simulink model "TricopterModel"  (R2015a)
settings: Solver=ode3  SolverMode=SingleTasking  StartTime=0.0  StopTime=10.0  FixedStep=T_sim  RelTol=1e-3
values from neighbouring files (symbols this model uses):
  a = 10.26    [SetupComplete.m]
  A_x = 0.015    [SetupComplete.m]
  A_y = A_x    (= 0.015)    [SetupComplete.m]
  A_z = 0.16    [SetupComplete.m]
  C_d0 = 0.001193    [SetupComplete.m]
  C_x = 1.2    [SetupComplete.m]
  C_y = C_x    (= 1.2)    [SetupComplete.m]
  C_z = 2.2    [SetupComplete.m]
  CG_0 = [0,0,0.02]'    [SetupComplete.m]
  eta_23 = deg2rad(-1.42)    [Run3Copter.m]
  h = 0.08    [SetupComplete.m]
  h_M = 0.064    [SetupComplete.m]
  I_BAC_0 = [ Ix,0,Ixz;0,Iy,0;Ixz,0,Iz]    [SetupComplete.m]
  Initial_Omegas = [1;1;1]*Omega_hover    [Run3Copter.m]
  l = 0.3450    (= 0.345)    [NDI_components.m]    (also in SetupComplete.m; robust_controller.m)
  l_arm = 0.264    [SetupComplete.m]
  m = 3.51    [SetupComplete.m]
  m_0 = 2.61    [SetupComplete.m]
  m_M = 0.300    (= 0.3)    [SetupComplete.m]
  R = 0.1778    [SetupComplete.m]    (also in robust_controller.m = eye(4))
  rho = 1.15    [SetupComplete.m]
  Rotation_sign = [ 1,-1,-1]    [SetupComplete.m]
  sigma = b*c/(pi*R)    (= 0.107416159567)    [SetupComplete.m]
  theta_0 = 0.38397    [SetupComplete.m]
  theta_1 = -0.2967    [SetupComplete.m]
  v_i0 = sqrt( 1/3*m*g/(2*rho*pi*R^2)  )    [SetupComplete.m]
undefined symbols (not defined in the file or in its folder): DOWN_0, EAST_0, Motor, NORTH_0, P_0, Prop, Q_0, R_0, Throttle_Hover, U_0, V_0, v_i_adim, Vx_adim, Vz_adim, W_0
undefined symbols (not defined in the file): Initial_Torques, J_FA, J_T, Tau_motors
libraries: XXCopter x22, simulink_extras x7, vrlib x6, XXCopter_C x3, aerolibutil x2, aerolib6dofsys x1
(part 1 of 2)
settings Model: ExtModeTrigDuration=5000  Creator=DavidTorres  LastModifiedBy=juan
settings OptimizationCC: BlockReduction=off  BooleanDataType=off
settings DebuggingCC: SaveWithParameterizedLinksMsg=none  UnderspecifiedInitializationDetection=Classic  MergeDetectMultiDrivingBlocksExec=none  SignalResolutionControl=TryResolveAllWithWarning
settings HardwareCC: TargetUnknown=on

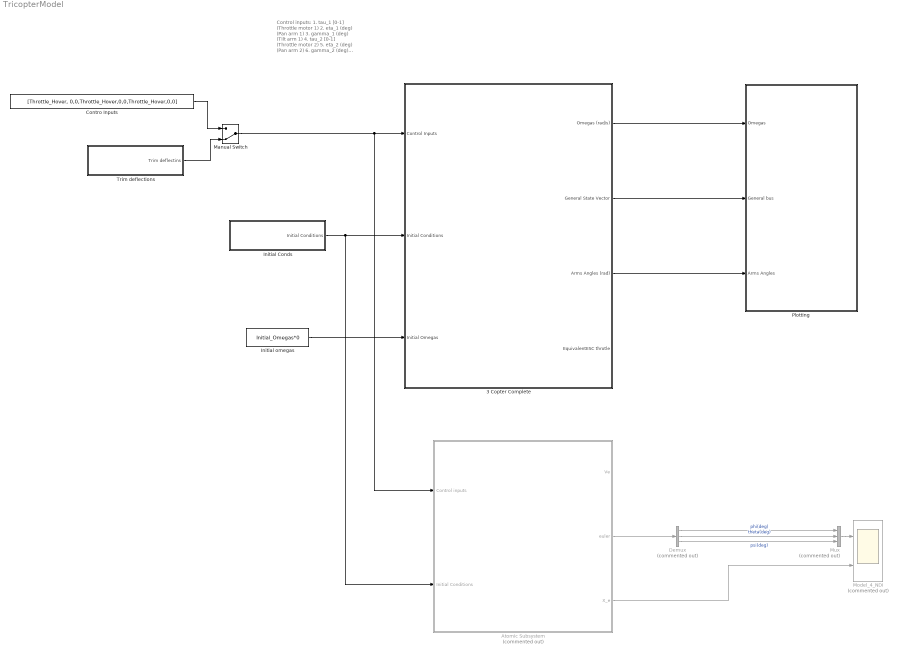
== system TricopterModel ==
  note: Control inputs:
      | 1. tau_1 [0-1] (Throttle motor 1)
      | 2. eta_1 (deg)  (Pan arm 1)
      | 3. gamma_1 (deg)  (Tilt arm 1)
      |
      | 4. tau_2 [0-1] (Throttle motor 2)
      | 5. eta_2 (deg)  (Pan arm 2)
      | 6. gamma_2 (deg)  (Tilt arm 2)
      |
      | 7. tau_3 [0-1] (Throttle motor 3)
      | 8. eta_3 (deg)  (Pan arm  3)
      | 9. gamma_3 (deg)  (Tilt arm 3)
  3 Copter Complete : Subsystem
  Atomic Subsystem : Subsystem  Commented=on
  Contro Inputs : Constant  Value=[Throttle_Hover, 0,0,Throttle_Hover,0,0,Throttle_Hover,0,0]
  Demux : Demux  Commented=on  Outputs=3
  Initial Conds : Subsystem  TreatAsAtomicUnit=on
  Initial omegas : Constant  Value=Initial_Omegas*0
  Manual Switch : ManualSwitch  CurrentSetting=0
  Model_4_NDI : Scope  Commented=on  NumInputPorts=2
      settings: ShowLegends=on  YMin=-5e-05~-21  YMax=0.00045~1  SaveName=ScopeData3
  Mux : Mux  Commented=on  Inputs=3
  Plotting : Subsystem
  Trim deflections : Subsystem  TreatAsAtomicUnit=on
  wires:
  Initial omegas/1 -> 3 Copter Complete/3(Initial Omegas)
  Initial Conds/1(Initial Conditions) -> Atomic Subsystem/2(Initial Conditions), 3 Copter Complete/2(Initial Conditions)
  3 Copter Complete/2(General State Vector) -> Plotting/2(General bus)
  3 Copter Complete/1(Omegas (rad/s)) -> Plotting/1(Omegas)
  3 Copter Complete/3(Arms Angles (rad)) -> Plotting/3(Arms Angles)
  Manual Switch/1 -> 3 Copter Complete/1(Control Inputs), Atomic Subsystem/1(Control inputs)
  Contro Inputs/1 -> Manual Switch/1
  Trim deflections/1(Trim deflectins) -> Manual Switch/2
  Atomic Subsystem/2(euler) -> Demux/1
  Demux/3 -> Mux/3  "psi(deg)"
  Demux/1 -> Mux/1  "phi(deg)"
  Demux/2 -> Mux/2  "theta(deg)"
  Mux/1 -> Model_4_NDI/1
  Atomic Subsystem/3(X_e) -> Model_4_NDI/2

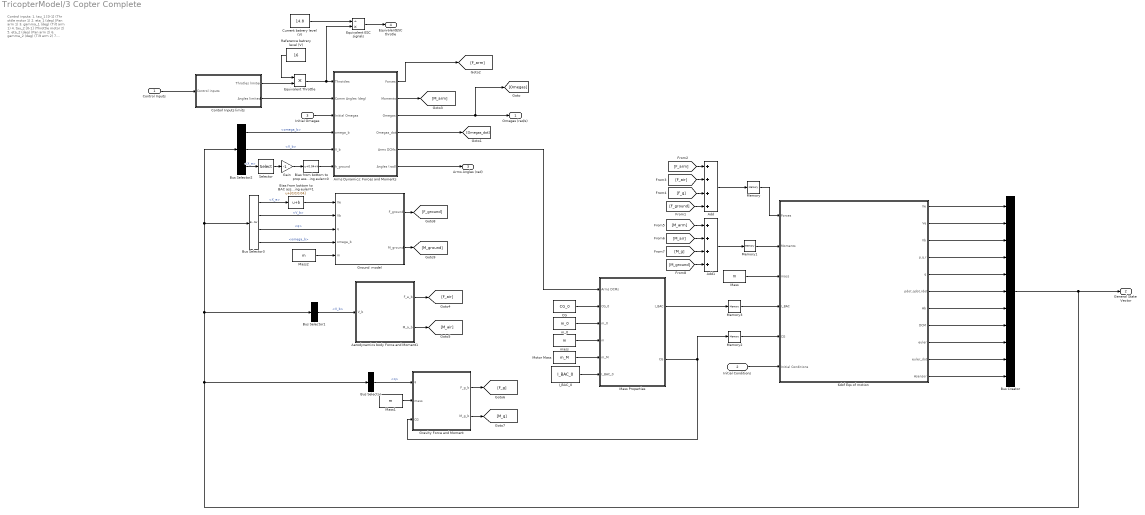
== system TricopterModel/3 Copter Complete ==
  note: Control inputs:
      | 1. tau_1 [0-1] (Thr ottle motor 1)
      | 2. eta_1 (deg)  (Pan arm 1)
      | 3. gamma_1 (deg)  (Tilt arm 1)
      |
      | 4. tau_2 [0-1] (Throttle motor 2)
      | 5. eta_2 (deg)  (Pan arm 2)
      | 6. gamma_2 (deg)  (Tilt arm 2)
      |
      | 7. tau_3 [0-1] (Throttle motor 3)
      | 8. eta_3 (deg)  (Pan arm  3)
      | 9. gamma_3 (deg)  (Tilt arm 3)
  Control Inputs : Inport
  Initial Conditions : Inport  Port=2
  Initial Omegas : Inport  Port=3
  6dof Eqs of motion : Subsystem  TreatAsAtomicUnit=on
  Add : Sum  Inputs=++++
  Add1 : Sum  Inputs=++++
  Aerodynamics body Force and Moment1 : MATLAB Function  TreatAsAtomicUnit=on
  Arms Dynamics: Forces and Moments : Subsystem
  Bias from bottom to BAC assuming euler=1 : Bias  Bias=[0;0;0.04]
  Bias from bottom to prop assuming euler=0 : Bias  Bias=0.04+h
  Bus Creator : BusCreator  Inputs=11
  Bus Selector : BusSelector  OutputSignals=q
  Bus Selector1 : BusSelector  OutputSignals=V_b
  Bus Selector2 : BusSelector  OutputSignals=omega_b,V_b,X_e
  Bus Selector3 : BusSelector  OutputSignals=X_e,V_b,q,omega_b
  CG : Constant  Value=CG_0
  Contorl Inputs limits : Subsystem  TreatAsAtomicUnit=on
  Current batrery level (V) : Constant  Value=14.8
  Equivalent ESC signals : Product  Inputs=/*
  Equivalent Throttle : Product  Inputs=**
  Gain : Gain  Gain=-1
  Gravity Force and Moment : MATLAB Function  TreatAsAtomicUnit=on
  Ground  model : Subsystem  TreatAsAtomicUnit=on
  I_BAC_0 : Constant  Value=I_BAC_0
  Mass : Constant  Value=m
  Mass Properties : Subsystem  TreatAsAtomicUnit=on
  Mass1 : Constant  Value=m
  Mass2 : Constant  Value=m
  Memory : Memory  X0=[0,0,0]
  Memory1 : Memory  X0=[0,0,0]
  Memory2 : Memory  X0=CG_0
  Memory3 : Memory  X0=I_BAC_0
  Motor Mass : Constant  Value=m_M
  Reference batrery level (V) : Constant  Value=16
  Selector : Selector  InputPortWidth=3  Indices=3
  m_0 : Constant  Value=m_0
  mass : Constant  Value=m
  Omegas (rad/s) : Outport
  General State Vector : Outport  Port=2
  Arms Angles (rad) : Outport  Port=3
  EquivalentESC throtle : Outport  Port=4
  wires:
  Initial Conditions/1 -> 6dof Eqs of motion/6(Initial Conditions)
  6dof Eqs of motion/3(Vb) -> Bus Creator/3
  6dof Eqs of motion/5(q) -> Bus Creator/5
  6dof Eqs of motion/2(Ve) -> Bus Creator/2
  6dof Eqs of motion/6(pdot,qdot,rdot) -> Bus Creator/6
  6dof Eqs of motion/1(Xe) -> Bus Creator/1
  6dof Eqs of motion/7(Ab) -> Bus Creator/7
  6dof Eqs of motion/8(DCM) -> Bus Creator/8
  6dof Eqs of motion/9(euler) -> Bus Creator/9
  6dof Eqs of motion/10(euler_dot) -> Bus Creator/10
  Bus Selector/1 -> Gravity Force and Moment/1(q)  "<q>"
  Mass/1 -> 6dof Eqs of motion/3(mass)
  Mass Properties/1(I_BAC) -> Memory3/1
  Bus Selector1/1 -> Aerodynamics body Force and Moment1/1(V_b)  "<V_b>"
  Bus Selector2/1 -> Arms Dynamics: Forces and Moments/4(omega_b)  "<omega_b>"
  Bus Selector2/2 -> Arms Dynamics: Forces and Moments/5(V_b)  "<V_b>"
  Mass1/1 -> Gravity Force and Moment/2(mass)
  Mass Properties/2(CG) -> Gravity Force and Moment/3(CG), Memory2/1
  Arms Dynamics: Forces and Moments/4(Omegas_dot) -> [Omegas_dot]
  Initial Omegas/1 -> Arms Dynamics: Forces and Moments/3(Initial Omegas)
  Bus Selector2/3 -> Selector/1  "<X_e>"
  Selector/1 -> Gain/1
  Gain/1 -> Bias from bottom to prop assuming euler=0/1
  Add/1 -> Memory/1
  Add1/1 -> Memory1/1
  Arms Dynamics: Forces and Moments/1(Forces) -> [F_arm]
  Arms Dynamics: Forces and Moments/2(Moments) -> [M_arm]
  Aerodynamics body Force and Moment1/1(F_a_b) -> [F_air]
  Aerodynamics body Force and Moment1/2(M_a_b) -> [M_air]
  Gravity Force and Moment/1(F_g_b) -> [F_g]
  Gravity Force and Moment/2(M_g_b) -> [M_g]
  [F_arm] -> Add/1
  [F_air] -> Add/2
  [F_g] -> Add/3
  [M_arm] -> Add1/1
  [M_g] -> Add1/3
  [M_air] -> Add1/2
  6dof Eqs of motion/11(Asensor) -> Bus Creator/11
  Contorl Inputs limits/1(Throtles limited) -> Equivalent Throttle/2
  Contorl Inputs limits/2(Angles limited) -> Arms Dynamics: Forces and Moments/2(Comm Angles (deg))
  Arms Dynamics: Forces and Moments/5(Arms DCMs) -> Mass Properties/1(Arms DCMs)
  CG/1 -> Mass Properties/2(CG_0)
  Motor Mass/1 -> Mass Properties/5(m_M)
  I_BAC_0/1 -> Mass Properties/6(I_BAC_0)
  m_0/1 -> Mass Properties/3(m_0)
  mass/1 -> Mass Properties/4(m)
  Arms Dynamics: Forces and Moments/3(Omegas) -> [Omegas], Omegas (rad/s)/1
  Bus Creator/1 -> Bus Selector2/1, Bus Selector3/1, Bus Selector1/1, Bus Selector/1, General State Vector/1
  Memory/1 -> 6dof Eqs of motion/1(Forces)
  Memory1/1 -> 6dof Eqs of motion/2(Moments)
  Memory2/1 -> 6dof Eqs of motion/5(CG)
  Memory3/1 -> 6dof Eqs of motion/4(I_BAC)
  Equivalent Throttle/1 -> Equivalent ESC signals/2, Arms Dynamics: Forces and Moments/1(Throttles)
  Reference batrery level (V)/1 -> Equivalent Throttle/1
  Current batrery level (V)/1 -> Equivalent ESC signals/1
  Equivalent ESC signals/1 -> EquivalentESC throtle/1
  6dof Eqs of motion/4(p,q,r) -> Bus Creator/4
  Arms Dynamics: Forces and Moments/6(Angles (rad)) -> Arms Angles (rad)/1
  Control Inputs/1 -> Contorl Inputs limits/1(Control inputs)
  Bus Selector3/1 -> Bias from bottom to BAC assuming euler=1/1  "<X_e>"
  Bus Selector3/3 -> Ground  model/3(q)  "<q>"
  Ground  model/1(F_ground) -> [F_ground]
  Ground  model/2(M_ground) -> [M_ground]
  [F_ground] -> Add/4
  [M_ground] -> Add1/4
  Mass2/1 -> Ground  model/5(m)
  Bus Selector3/2 -> Ground  model/2(Vb)  "<V_b>"
  Bus Selector3/4 -> Ground  model/4(omega_b)  "<omega_b>"
  Bias from bottom to prop assuming euler=0/1 -> Arms Dynamics: Forces and Moments/6(h_ground)
  Bias from bottom to BAC assuming euler=1/1 -> Ground  model/1(Xe)

== system TricopterModel/Atomic Subsystem ==
  Control inputs : Inport
  Initial Conditions : Inport  Port=2
  3Copter_4_NDI : Subsystem
  Bus Selector : BusSelector  OutputSignals=X_e_0,V_e_0,Euler_0,Euler_dot_0
  Ground : Ground
  Ground1 : Ground
  Ground2 : Ground
  Normalize Quaternion : Subsystem  TreatAsAtomicUnit=on
  SVFI_to_SVFb : MATLAB Function  TreatAsAtomicUnit=on
  SV_F_b_to_SV_FI : MATLAB Function  TreatAsAtomicUnit=on
  "p,q,r " : Integrator  InitialConditionSource=external  InitialCondition=[P_0,Q_0,R_0]
  quaternion : Integrator  InitialConditionSource=external  InitialCondition=[P_0,Q_0,R_0]
  ub,vb,wb : Integrator  InitialConditionSource=external  InitialCondition=[U_0,V_0,W_0]
  xe,ye,ze : Integrator  InitialConditionSource=external  InitialCondition=[NORTH_0,EAST_0,-DOWN_0]
  Ve : Outport
  euler : Outport  Port=2
  X_e : Outport  Port=3
  wires:
  Initial Conditions/1 -> Bus Selector/1
  Bus Selector/1 -> SVFI_to_SVFb/1(X_e)  "<X_e_0>"
  Bus Selector/2 -> SVFI_to_SVFb/2(V_e)  "<V_e_0>"
  Bus Selector/3 -> SVFI_to_SVFb/3(Euler_Ang)  "<Euler_0>"
  Bus Selector/4 -> SVFI_to_SVFb/4(Euler_Ang_Dot)  "<Euler_dot_0>"
  3Copter_4_NDI/4(omega_b_dot) -> "p,q,r "/1
  SVFI_to_SVFb/4(omega_b) -> "p,q,r "/2
  3Copter_4_NDI/3(q_dot) -> quaternion/1
  SVFI_to_SVFb/3(q) -> quaternion/2
  quaternion/1 -> Normalize Quaternion/1(q)
  3Copter_4_NDI/2(Ab) -> ub,vb,wb/1
  SVFI_to_SVFb/2(V_b) -> ub,vb,wb/2
  3Copter_4_NDI/1(Ve) -> Ve/1, xe,ye,ze/1
  Control inputs/1 -> 3Copter_4_NDI/1(Control Inputs)
  SVFI_to_SVFb/1(X_e_out) -> xe,ye,ze/2
  xe,ye,ze/1 -> X_e/1, 3Copter_4_NDI/2(X_e)
  ub,vb,wb/1 -> 3Copter_4_NDI/3(Vb)
  Normalize Quaternion/1(normal(q)) -> SV_F_b_to_SV_FI/1(q), 3Copter_4_NDI/4(q)
  "p,q,r "/1 -> 3Copter_4_NDI/5(omega_b)
  Ground/1 -> 3Copter_4_NDI/6(Omegas_dot_actual)
  Ground1/1 -> 3Copter_4_NDI/7(angles_actual)
  Ground2/1 -> 3Copter_4_NDI/8(angles_dot_actual)
  SV_F_b_to_SV_FI/1(euler) -> euler/1  "euler"

== system TricopterModel/Initial Conds ==
  Bus Creator : BusCreator
  Ini Position X_e_0 : Constant  Value=[0;0;-1]
  Initial Attitude Euler_0 : Constant  Value=[deg2rad(0);deg2rad(0);deg2rad(0)]
  Initial Attitude Rate  Euler_dot_0 : Constant  Value=[deg2rad(0);deg2rad(0);deg2rad(0)]
  Initial Velocity V_e_0 : Constant  Value=[0;0;0]
  Initial Conditions : Outport
  wires:
  Ini Position X_e_0/1 -> Bus Creator/1  "X_e_0"
  Initial Velocity V_e_0/1 -> Bus Creator/2  "V_e_0"
  Initial Attitude Euler_0/1 -> Bus Creator/3  "Euler_0"
  Initial Attitude Rate  Euler_dot_0/1 -> Bus Creator/4  "Euler_dot_0"
  Bus Creator/1 -> Initial Conditions/1

== system TricopterModel/Plotting ==
  Omegas : Inport
  General bus : Inport  Port=2
  Arms Angles : Inport  Port=3
  Bus Selector : BusSelector  OutputSignals=euler,X_e,DCM
  Bus Selector1 : BusSelector  OutputSignals=Angles Arm 1,Angles Arm 2,Angles Arm 3
  Demux : Demux  Outputs=3
  Level-2 MATLAB S-Function : M-S-Function  FunctionName=Simulation_3_copter
  Mux : Mux  Inputs=3
  Scope : Scope  NumInputPorts=2
      settings: ShowLegends=on  YMin=-5e-05~-21  YMax=0.00045~1
  Scope1 : Scope
      settings: TimeRange=5  YMin=564.75  YMax=570
  Scope2 : Scope  NumInputPorts=3
      settings: ShowLegends=on  YMin=-5~-5~-5  YMax=5~5~5  SaveName=ScopeData2
  wires:
  General bus/1 -> Bus Selector/1
  Bus Selector/1 -> Demux/1  "<euler>"
  Omegas/1 -> Scope1/1  "Omegas"
  Arms Angles/1 -> Bus Selector1/1
  Bus Selector1/3 -> Level-2 MATLAB S-Function/8, Scope2/3  "<Angles Arm 3>"
  Bus Selector1/2 -> Level-2 MATLAB S-Function/7, Scope2/2  "<Angles Arm 2>"
  Bus Selector1/1 -> Level-2 MATLAB S-Function/6, Scope2/1  "<Angles Arm 1>"
  Bus Selector/2 -> Level-2 MATLAB S-Function/1, Scope/2  "<X_e>"
  [r_p_3] -> Level-2 MATLAB S-Function/5
  [r_p_2] -> Level-2 MATLAB S-Function/4
  [r_p_1] -> Level-2 MATLAB S-Function/3
  Bus Selector/3 -> Level-2 MATLAB S-Function/2  "<DCM>"
  Demux/3 -> Mux/3  "psi(deg)"
  Demux/1 -> Mux/1  "phi(deg)"
  Demux/2 -> Mux/2  "theta(deg)"
  Mux/1 -> Scope/1

== system TricopterModel/Trim deflections ==
  " " : simulink_extras/Transformations/Radians to Degrees
  Contro Inputs1 : Constant  Value=0
  Contro Inputs2 : Constant  Value=0
  Contro Inputs3 : Constant  Value=eta_23
  Gain : Gain  Gain=-1
  Ground : Ground
  Mux : Mux  Inputs=9
  Trim deflectins : Outport
  wires:
  Contro Inputs1/1 -> Mux/1
  Contro Inputs2/1 -> Mux/7, Mux/4
  Ground/1 -> Mux/2, Mux/6, Mux/9, Mux/3
  Contro Inputs3/1 -> " "/1
  " "/1 -> Gain/1, Mux/5
  Gain/1 -> Mux/8
  Mux/1 -> Trim deflectins/1

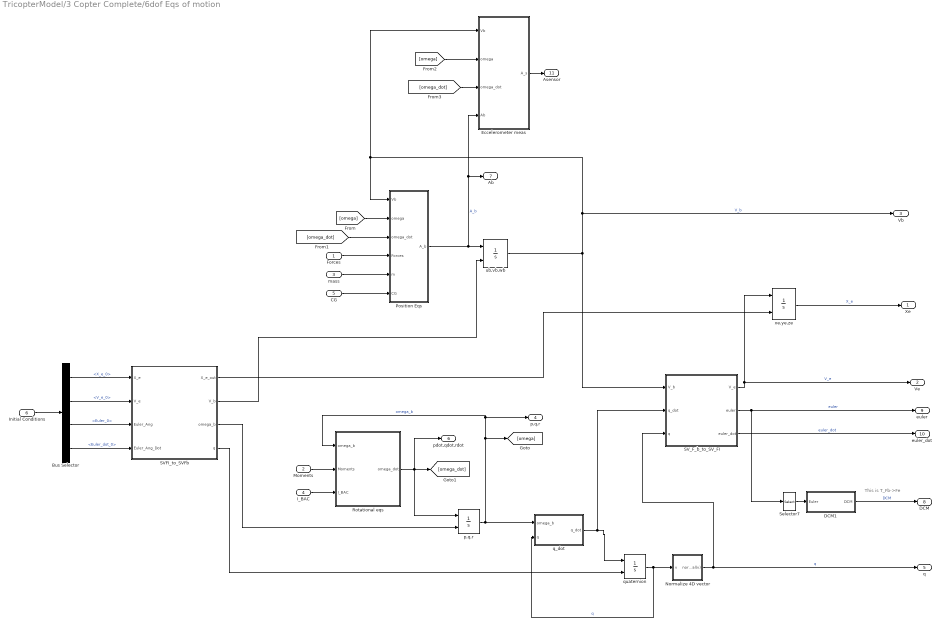
== system TricopterModel/3 Copter Complete/6dof Eqs of motion ==
  note: This is T_Fb->Fe
  Forces : Inport
  Moments : Inport  Port=2
  mass : Inport  Port=3
  I_BAC : Inport  Port=4
  CG : Inport  Port=5
  Initial Conditions : Inport  Port=6
  Bus Selector : BusSelector  OutputSignals=X_e_0,V_e_0,Euler_0,Euler_dot_0
  DCM1 : Subsystem  TreatAsAtomicUnit=on
  Eccelerometer meas : MATLAB Function  TreatAsAtomicUnit=on
  Normalize 4D vector : Subsystem  AncestorBlock=XXCopter/Normalize 4D vector  TreatAsAtomicUnit=on
  Position Eqs : MATLAB Function  TreatAsAtomicUnit=on
  Rotational eqs : MATLAB Function  TreatAsAtomicUnit=on
  SVFI_to_SVFb : MATLAB Function  TreatAsAtomicUnit=on
  SV_F_b_to_SV_FI : MATLAB Function  TreatAsAtomicUnit=on
  Selector7 : Selector  InputPortWidth=3  Indices=[3 2 1]
  "p,q,r " : Integrator  InitialConditionSource=external  InitialCondition=[P_0,Q_0,R_0]
  q_dot : Subsystem  TreatAsAtomicUnit=on
  quaternion : Integrator  InitialConditionSource=external  InitialCondition=[P_0,Q_0,R_0]
  ub,vb,wb : Integrator  InitialConditionSource=external  InitialCondition=[U_0,V_0,W_0]
  xe,ye,ze : Integrator  InitialConditionSource=external  InitialCondition=[NORTH_0,EAST_0,-DOWN_0]
  Xe : Outport
  Ve : Outport  Port=2
  Vb : Outport  Port=3
  p,q,r : Outport  Port=4
  q : Outport  Port=5
  pdot,qdot,rdot : Outport  Port=6
  Ab : Outport  Port=7
  DCM : Outport  Port=8
  euler : Outport  Port=9
  euler_dot : Outport  Port=10
  Asensor : Outport  Port=11
  wires:
  I_BAC/1 -> Rotational eqs/3(I_BAC)
  mass/1 -> Position Eqs/5(m)
  Forces/1 -> Position Eqs/4(Forces)
  xe,ye,ze/1 -> Xe/1  "X_e"
  ub,vb,wb/1 -> Vb/1, Eccelerometer meas/1(Vb), Position Eqs/1(Vb), SV_F_b_to_SV_FI/1(V_b)  "V_b"
  SV_F_b_to_SV_FI/1(V_e) -> Ve/1, xe,ye,ze/1  "V_e"
  [omega] -> Position Eqs/2(omega)
  [omega_dot] -> Position Eqs/3(omega_dot)
  Position Eqs/1(A_b) -> Eccelerometer meas/4(Ab), Ab/1, ub,vb,wb/1  "A_b"
  CG/1 -> Position Eqs/6(CG)
  Initial Conditions/1 -> Bus Selector/1
  Bus Selector/1 -> SVFI_to_SVFb/1(X_e)  "<X_e_0>"
  Bus Selector/2 -> SVFI_to_SVFb/2(V_e)  "<V_e_0>"
  Bus Selector/3 -> SVFI_to_SVFb/3(Euler_Ang)  "<Euler_0>"
  Bus Selector/4 -> SVFI_to_SVFb/4(Euler_Ang_Dot)  "<Euler_dot_0>"
  SVFI_to_SVFb/2(V_b) -> ub,vb,wb/2
  SVFI_to_SVFb/1(X_e_out) -> xe,ye,ze/2
  SVFI_to_SVFb/3(omega_b) -> "p,q,r "/2
  Rotational eqs/1(omega_dot) -> pdot,qdot,rdot/1, [omega_dot], "p,q,r "/1
  "p,q,r "/1 -> q_dot/1(omega_b), [omega], p,q,r/1, Rotational eqs/1(omega_b)  "omega_b"
  q_dot/1(q_dot) -> quaternion/1, SV_F_b_to_SV_FI/2(q_dot)
  SVFI_to_SVFb/4(q) -> quaternion/2
  quaternion/1 -> Normalize 4D vector/1(v), q_dot/2(q)  "q"
  SV_F_b_to_SV_FI/2(euler) -> Selector7/1, euler/1  "euler"
  SV_F_b_to_SV_FI/3(euler_dot) -> euler_dot/1  "euler_dot"
  Moments/1 -> Rotational eqs/2(Moments)
  Normalize 4D vector/1(normal(v)) -> q/1, SV_F_b_to_SV_FI/3(q)  "q"
  [omega] -> Eccelerometer meas/2(omega)
  [omega_dot] -> Eccelerometer meas/3(omega_dot)
  Eccelerometer meas/1(A_s) -> Asensor/1
  DCM1/1(DCM) -> DCM/1  "DCM"
  Selector7/1 -> DCM1/1(Euler)

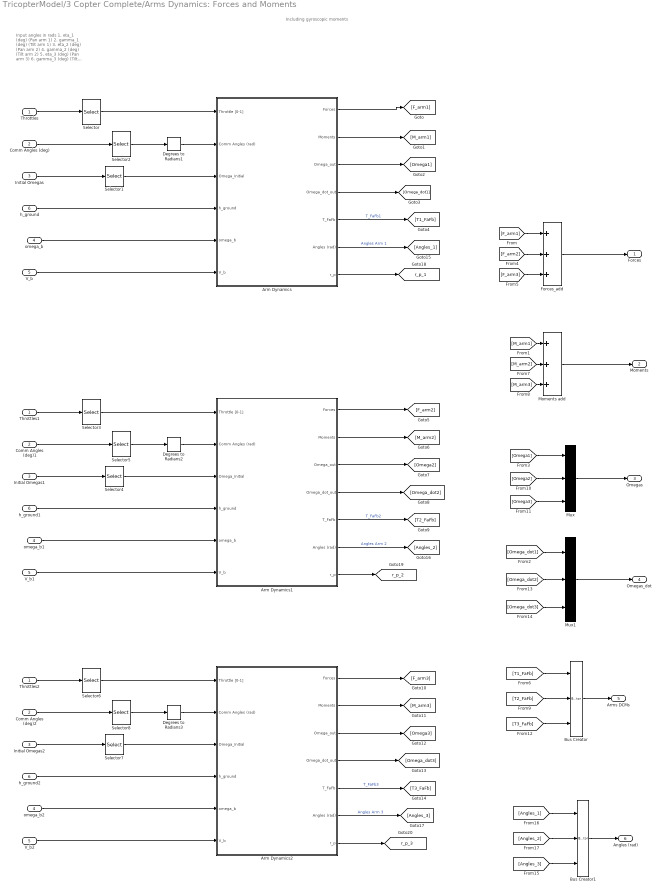
== system TricopterModel/3 Copter Complete/Arms Dynamics: Forces and Moments ==
  note: Including gyroscopic moments
  note: Input angles in rads
      |
      | 1. eta_1 (deg)  (Pan arm 1)
      | 2. gamma_1 (deg)  (Tilt arm 1)
      |
      | 3. eta_2 (deg)  (Pan arm 2)
      | 4. gamma_2 (deg)  (Tilt arm 2)
      |
      | 5. eta_3 (deg)  (Pan arm  3)
      | 6. gamma_3 (deg)  (Tilt arm 3)
  Throttles : Inport
  Comm Angles (deg) : Inport  Port=2
  Initial Omegas : Inport  Port=3
  omega_b : Inport  Port=4
  V_b : Inport  Port=5
  h_ground : Inport  Port=6
  Arm Dynamics : Subsystem  AncestorBlock=XXCopter/Arm Dynamics  TreatAsAtomicUnit=on  mask(Arm dynamics, kinematics, forces and moments){Rot_sign=Rotation_sign(1), tau=Tau_motors, arm_hub_pos=l*[1;0;0], arm_axis=[l_arm;0;0], arm_num=1, eta_dir=[1;0;0], gamma_dir=[0;1;0], J_T=J_T, J_FA=J_FA, h=h, Torq_ini=Initial_Torques(1), Omega_ini=Initial_Omegas(1), init_eta=0, init_gamma=0, omega_n=35, xi=1.45, c=0}
      mask prompts: Rot_sign "Rotation sign"; tau "Tau motors"; arm_hub_pos "Arm Hub position"; arm_axis "Arm Hub from servo"; arm_num "Arm number"; eta_dir "eta direcction"; gamma_dir "gamma direction"; J_T "Inertia Motor+prop"; J_FA "Inertia Forearm"; h "h propeller hub"; Torq_ini "Torque Initial Condition"; Omega_ini "Omega Initial Condition"; init_eta "Initial eta  (rad)"; init_gamma "Initial gamma  (rad)"; omega_n "Servo natural frequency"; xi "Servo damping"; c "Derivative param"
      mask help:
      | This block only accepts arms oriented in x-axis or y-axis: eta and gamma directions can only be [1,0,0] or [0,1,0]
      | Note rotations order is [eta (pan) ,gamma (tilt),0]
      |
      | If Arm number 1 (Forward one)
      | eta_dir=[1,0,0]
      | gamma_dir=[0,1,0]
      |
      | If Arm number 2 or 3 (rear ones)
      | eta_dir=[0,1,0]
      | gamma_dir=[1,0,0]
      mask TypeOptions Rot_sign: Aerodynamics Propeller/Rot_sign | Gyroscopic Moments/Rot_sign
      mask TypeOptions tau: ESC+Motor Dynamcis/tau
      mask TypeOptions arm_hub_pos: Arms Kinematics/Arm_hub_position
      mask TypeOptions arm_axis: Gyroscopic Moments/Arm_axis
      mask TypeOptions arm_num: Arms Kinematics/Arm_number
      mask TypeOptions eta_dir: Arms Kinematics/eta_dir | Gyroscopic Moments/eta_dir
      mask TypeOptions gamma_dir: Arms Kinematics/gamma_dir | Gyroscopic Moments/gamma_dir
      mask TypeOptions J_T: ESC+Motor Dynamcis/J_T | Gyroscopic Moments/J_T
      mask TypeOptions J_FA: Gyroscopic Moments/J_FA
      mask TypeOptions h: Arms Kinematics/h_prop
      mask TypeOptions Torq_ini: Initial_torque/X0
      mask TypeOptions Omega_ini: initial_omega/X0
      mask TypeOptions init_eta: Servos Dynamics/init_eta
      mask TypeOptions omega_n: Servos Dynamics/omega_n
      mask TypeOptions xi: Servos Dynamics/xi
      mask TypeOptions c: Servos Dynamics/derv_param
      mask Display:
      | % fprintf(' Arm number %i \n dynamics',arm_num)
      | 
      | 
      | disp(['{\bf \fontsize{16}',sprintf('Arm number\n\n'),num2str(arm_num),sprintf('\n\n Dynamics '),'}'], 'texmode','on');
  Arm Dynamics1 : Subsystem  AncestorBlock=XXCopter/Arm Dynamics  TreatAsAtomicUnit=on  mask(Arm dynamics, kinematics, forces and moments){Rot_sign=Rotation_sign(2), tau=Tau_motors, arm_hub_pos=l*[-1/2;sqrt(3)/2;0], arm_axis=[0;l_arm;0], arm_num=2, eta_dir=[0;1;0], gamma_dir=[1;0;0], J_T=J_T, J_FA=J_FA, h=h, Torq_ini=Initial_Torques(2), Omega_ini=Initial_Omegas(2), init_eta=0, init_gamma=0, omega_n=35, xi=1.45, c=0}
      mask prompts: Rot_sign "Rotation sign"; tau "Tau motors"; arm_hub_pos "Arm Hub position"; arm_axis "Arm Hub from servo"; arm_num "Arm number"; eta_dir "eta direcction"; gamma_dir "gamma direction"; J_T "Inertia Motor+prop"; J_FA "Inertia Forearm"; h "h propeller hub"; Torq_ini "Torque Initial Condition"; Omega_ini "Omega Initial Condition"; init_eta "Initial eta  (rad)"; init_gamma "Initial gamma  (rad)"; omega_n "Servo natural frequency"; xi "Servo damping"; c "Derivative param"
      mask help:
      | This block only accepts arms oriented in x-axis or y-axis: eta and gamma directions can only be [1,0,0] or [0,1,0]
      | Note rotations order is [eta (pan) ,gamma (tilt),0]
      |
      | If Arm number 1 (Forward one)
      | eta_dir=[1,0,0]
      | gamma_dir=[0,1,0]
      |
      | If Arm number 2 or 3 (rear ones)
      | eta_dir=[0,1,0]
      | gamma_dir=[1,0,0]
      mask TypeOptions Rot_sign: Aerodynamics Propeller/Rot_sign | Gyroscopic Moments/Rot_sign
      mask TypeOptions tau: ESC+Motor Dynamcis/tau
      mask TypeOptions arm_hub_pos: Arms Kinematics/Arm_hub_position
      mask TypeOptions arm_axis: Gyroscopic Moments/Arm_axis
      mask TypeOptions arm_num: Arms Kinematics/Arm_number
      mask TypeOptions eta_dir: Arms Kinematics/eta_dir | Gyroscopic Moments/eta_dir
      mask TypeOptions gamma_dir: Arms Kinematics/gamma_dir | Gyroscopic Moments/gamma_dir
      mask TypeOptions J_T: ESC+Motor Dynamcis/J_T | Gyroscopic Moments/J_T
      mask TypeOptions J_FA: Gyroscopic Moments/J_FA
      mask TypeOptions h: Arms Kinematics/h_prop
      mask TypeOptions Torq_ini: Initial_torque/X0
      mask TypeOptions Omega_ini: initial_omega/X0
      mask TypeOptions init_eta: Servos Dynamics/init_eta
      mask TypeOptions omega_n: Servos Dynamics/omega_n
      mask TypeOptions xi: Servos Dynamics/xi
      mask TypeOptions c: Servos Dynamics/derv_param
      mask Display:
      | % fprintf(' Arm number %i \n dynamics',arm_num)
      | 
      | 
      | disp(['{\bf \fontsize{16}',sprintf('Arm number\n\n'),num2str(arm_num),sprintf('\n\n Dynamics '),'}'], 'texmode','on');
  Arm Dynamics2 : Subsystem  AncestorBlock=XXCopter/Arm Dynamics  TreatAsAtomicUnit=on  mask(Arm dynamics, kinematics, forces and moments){Rot_sign=Rotation_sign(3), tau=Tau_motors, arm_hub_pos=l*[-1/2;-sqrt(3)/2;0], arm_axis=[0;-l_arm;0], arm_num=3, eta_dir=[0;1;0], gamma_dir=[1;0;0], J_T=J_T, J_FA=J_FA, h=h, Torq_ini=Initial_Torques(3), Omega_ini=Initial_Omegas(3), init_eta=0, init_gamma=0, omega_n=35, xi=1.45, c=0}
      mask prompts: Rot_sign "Rotation sign"; tau "Tau motors"; arm_hub_pos "Arm Hub position"; arm_axis "Arm Hub from servo"; arm_num "Arm number"; eta_dir "eta direcction"; gamma_dir "gamma direction"; J_T "Inertia Motor+prop"; J_FA "Inertia Forearm"; h "h propeller hub"; Torq_ini "Torque Initial Condition"; Omega_ini "Omega Initial Condition"; init_eta "Initial eta  (rad)"; init_gamma "Initial gamma  (rad)"; omega_n "Servo natural frequency"; xi "Servo damping"; c "Derivative param"
      mask help:
      | This block only accepts arms oriented in x-axis or y-axis: eta and gamma directions can only be [1,0,0] or [0,1,0]
      | Note rotations order is [eta (pan) ,gamma (tilt),0]
      |
      | If Arm number 1 (Forward one)
      | eta_dir=[1,0,0]
      | gamma_dir=[0,1,0]
      |
      | If Arm number 2 or 3 (rear ones)
      | eta_dir=[0,1,0]
      | gamma_dir=[1,0,0]
      mask TypeOptions Rot_sign: Aerodynamics Propeller/Rot_sign | Gyroscopic Moments/Rot_sign
      mask TypeOptions tau: ESC+Motor Dynamcis/tau
      mask TypeOptions arm_hub_pos: Arms Kinematics/Arm_hub_position
      mask TypeOptions arm_axis: Gyroscopic Moments/Arm_axis
      mask TypeOptions arm_num: Arms Kinematics/Arm_number
      mask TypeOptions eta_dir: Arms Kinematics/eta_dir | Gyroscopic Moments/eta_dir
      mask TypeOptions gamma_dir: Arms Kinematics/gamma_dir | Gyroscopic Moments/gamma_dir
      mask TypeOptions J_T: ESC+Motor Dynamcis/J_T | Gyroscopic Moments/J_T
      mask TypeOptions J_FA: Gyroscopic Moments/J_FA
      mask TypeOptions h: Arms Kinematics/h_prop
      mask TypeOptions Torq_ini: Initial_torque/X0
      mask TypeOptions Omega_ini: initial_omega/X0
      mask TypeOptions init_eta: Servos Dynamics/init_eta
      mask TypeOptions omega_n: Servos Dynamics/omega_n
      mask TypeOptions xi: Servos Dynamics/xi
      mask TypeOptions c: Servos Dynamics/derv_param
      mask Display:
      | % fprintf(' Arm number %i \n dynamics',arm_num)
      | 
      | 
      | disp(['{\bf \fontsize{16}',sprintf('Arm number\n\n'),num2str(arm_num),sprintf('\n\n Dynamics '),'}'], 'texmode','on');
  Bus Creator : BusCreator  Inputs=3
  Bus Creator1 : BusCreator  Inputs=3
  Comm Angles (deg)1 : InportShadow  Port=2
  Comm Angles (deg)2 : InportShadow  Port=2
  Degrees to Radians1 : simulink_extras/Transformations/Degrees to Radians
  Degrees to Radians2 : simulink_extras/Transformations/Degrees to Radians
  Degrees to Radians3 : simulink_extras/Transformations/Degrees to Radians
  Forces_add : Sum  Inputs=+++
  Initial Omegas1 : InportShadow  Port=3
  Initial Omegas2 : InportShadow  Port=3
  Moments add : Sum  Inputs=+++
  Mux : Mux  Inputs=3
  Mux1 : Mux  Inputs=3
  Selector : Selector  InputPortWidth=3  Indices=[1]
  Selector1 : Selector  InputPortWidth=3  Indices=[1]
  Selector2 : Selector  InputPortWidth=6  Indices=[1,2]
  Selector3 : Selector  InputPortWidth=3  Indices=2
  Selector4 : Selector  InputPortWidth=3  Indices=2
  Selector5 : Selector  InputPortWidth=6  Indices=[3,4]
  Selector6 : Selector  InputPortWidth=3  Indices=3
  Selector7 : Selector  InputPortWidth=3  Indices=3
  Selector8 : Selector  InputPortWidth=6  Indices=[5,6]
  Throttles1 : InportShadow
  Throttles2 : InportShadow
  V_b1 : InportShadow  Port=5
  V_b2 : InportShadow  Port=5
  h_ground1 : InportShadow  Port=6
  h_ground2 : InportShadow  Port=6
  omega_b1 : InportShadow  Port=4
  omega_b2 : InportShadow  Port=4
  Forces : Outport
  Moments : Outport  Port=2
  Omegas : Outport  Port=3
  Omegas_dot : Outport  Port=4
  Arms DCMs : Outport  Port=5
  Angles (rad) : Outport  Port=6
  tag scope: r_p_1=global, r_p_2=global, r_p_3=global
  wires:
  Selector1/1 -> Arm Dynamics/3(Omega_Initial)
  Throttles/1 -> Selector/1
  Initial Omegas/1 -> Selector1/1
  Selector/1 -> Arm Dynamics/1(Throttle [0-1])
  V_b/1 -> Arm Dynamics/6(V_b)
  Forces_add/1 -> Forces/1
  Moments add/1 -> Moments/1
  Mux/1 -> Omegas/1
  Mux1/1 -> Omegas_dot/1
  h_ground/1 -> Arm Dynamics/4(h_ground)
  Arm Dynamics/1(Forces) -> [F_arm1]
  Arm Dynamics/2(Moments) -> [M_arm1]
  Arm Dynamics/3(Omega_out) -> [Omega1]
  Arm Dynamics/4(Omega_dot_out) -> [Omega_dot1]
  [F_arm1] -> Forces_add/1
  [M_arm1] -> Moments add/1
  [Omega_dot1] -> Mux1/1
  [Omega1] -> Mux/1
  omega_b/1 -> Arm Dynamics/5(omega_b)
  [F_arm2] -> Forces_add/2
  [F_arm3] -> Forces_add/3
  [Omega2] -> Mux/2
  [Omega3] -> Mux/3
  [Omega_dot2] -> Mux1/2
  [Omega_dot3] -> Mux1/3
  [M_arm3] -> Moments add/3
  [M_arm2] -> Moments add/2
  Degrees to Radians1/1 -> Arm Dynamics/2(Comm Angles (rad))
  Comm Angles (deg)/1 -> Selector2/1
  Selector2/1 -> Degrees to Radians1/1
  Arm Dynamics/5(T_FaFb) -> [T1_FaFb]  "T_FaFb1"
  Bus Creator/1 -> Arms DCMs/1
  [T1_FaFb] -> Bus Creator/1
  Selector4/1 -> Arm Dynamics1/3(Omega_Initial)
  Throttles1/1 -> Selector3/1
  Initial Omegas1/1 -> Selector4/1
  Selector3/1 -> Arm Dynamics1/1(Throttle [0-1])
  V_b1/1 -> Arm Dynamics1/6(V_b)
  h_ground1/1 -> Arm Dynamics1/4(h_ground)
  Arm Dynamics1/1(Forces) -> [F_arm2]
  Arm Dynamics1/2(Moments) -> [M_arm2]
  Arm Dynamics1/3(Omega_out) -> [Omega2]
  Arm Dynamics1/4(Omega_dot_out) -> [Omega_dot2]
  omega_b1/1 -> Arm Dynamics1/5(omega_b)
  Degrees to Radians2/1 -> Arm Dynamics1/2(Comm Angles (rad))
  Comm Angles (deg)1/1 -> Selector5/1
  Selector5/1 -> Degrees to Radians2/1
  Arm Dynamics1/5(T_FaFb) -> [T2_FaFb]  "T_FaFb2"
  [T2_FaFb] -> Bus Creator/2
  Selector7/1 -> Arm Dynamics2/3(Omega_Initial)
  Throttles2/1 -> Selector6/1
  Initial Omegas2/1 -> Selector7/1
  Selector6/1 -> Arm Dynamics2/1(Throttle [0-1])
  V_b2/1 -> Arm Dynamics2/6(V_b)
  h_ground2/1 -> Arm Dynamics2/4(h_ground)
  Arm Dynamics2/1(Forces) -> [F_arm3]
  Arm Dynamics2/2(Moments) -> [M_arm3]
  Arm Dynamics2/3(Omega_out) -> [Omega3]
  Arm Dynamics2/4(Omega_dot_out) -> [Omega_dot3]
  omega_b2/1 -> Arm Dynamics2/5(omega_b)
  Degrees to Radians3/1 -> Arm Dynamics2/2(Comm Angles (rad))
  Comm Angles (deg)2/1 -> Selector8/1
  Selector8/1 -> Degrees to Radians3/1
  Arm Dynamics2/5(T_FaFb) -> [T3_FaFb]  "T_FaFb3"
  [T3_FaFb] -> Bus Creator/3
  Bus Creator1/1 -> Angles (rad)/1
  [Angles_1] -> Bus Creator1/1
  [Angles_2] -> Bus Creator1/2
  [Angles_3] -> Bus Creator1/3
  Arm Dynamics/6(Angles (rad)) -> [Angles_1]  "Angles Arm 1"
  Arm Dynamics1/6(Angles (rad)) -> [Angles_2]  "Angles Arm 2"
  Arm Dynamics2/6(Angles (rad)) -> [Angles_3]  "Angles Arm 3"
  Arm Dynamics/7(r_p) -> [r_p_1]
  Arm Dynamics1/7(r_p) -> [r_p_2]
  Arm Dynamics2/7(r_p) -> [r_p_3]

== system TricopterModel/3 Copter Complete/Contorl Inputs limits ==
  note: limits in degs
  Control inputs : Inport
  Demux : Demux  Outputs=6
  Mux : Mux  Inputs=6
  Saturation : Saturate  UpperLimit=1  LowerLimit=0
  Throttles : Selector  InputPortWidth=9  Indices=[1,4,7]
  "angles " : Selector  InputPortWidth=9  Indices=[2,3,5,6,8,9]
  eta 1 : Saturate  UpperLimit=180  LowerLimit=-180
  eta 2 : Saturate  UpperLimit=180  LowerLimit=-180
  eta 3 : Saturate  UpperLimit=180  LowerLimit=-180
  gamma 2 : Saturate  UpperLimit=90  LowerLimit=-30
  gamma1 : Saturate  UpperLimit=30  LowerLimit=-90
  gamma3 : Saturate  UpperLimit=30  LowerLimit=-90
  Throtles limited : Outport
  Angles limited : Outport  Port=2
  wires:
  Control inputs/1 -> Throttles/1, "angles "/1
  Throttles/1 -> Saturation/1
  "angles "/1 -> Demux/1
  Demux/1 -> eta 1/1
  Demux/2 -> gamma1/1
  Demux/3 -> eta 2/1
  Demux/4 -> gamma 2/1
  Demux/5 -> eta 3/1
  Demux/6 -> gamma3/1
  eta 1/1 -> Mux/1
  gamma1/1 -> Mux/2
  eta 2/1 -> Mux/3
  gamma 2/1 -> Mux/4
  eta 3/1 -> Mux/5
  gamma3/1 -> Mux/6
  Mux/1 -> Angles limited/1
  Saturation/1 -> Throtles limited/1

== system TricopterModel/3 Copter Complete/Ground  model ==
  Xe : Inport
  Vb : Inport  Port=2
  q : Inport  Port=3
  omega_b : Inport  Port=4
  m : Inport  Port=5
  Ground model logic and Forces and moments : MATLAB Function  TreatAsAtomicUnit=on
  arm_hub position 1 : Constant  Value=l*[1;0;0]
  arm_hub position 2 : Constant  Value=l*[-1/2;sqrt(3)/2;0]
  arm_hub position 3 : Constant  Value=l*[-1/2;-sqrt(3)/2;0]
  F_ground : Outport
  M_ground : Outport  Port=2
  wires:
  Xe/1 -> Ground model logic and Forces and moments/1(Xe)
  q/1 -> Ground model logic and Forces and moments/3(q)
  m/1 -> Ground model logic and Forces and moments/5(mass)
  arm_hub position 1/1 -> Ground model logic and Forces and moments/6(Arm1)
  arm_hub position 2/1 -> Ground model logic and Forces and moments/7(Arm2)
  arm_hub position 3/1 -> Ground model logic and Forces and moments/8(Arm3)
  Ground model logic and Forces and moments/2(M_gr_b) -> M_ground/1
  Ground model logic and Forces and moments/1(F_gr_b) -> F_ground/1
  Vb/1 -> Ground model logic and Forces and moments/2(Vb)
  omega_b/1 -> Ground model logic and Forces and moments/4(omega_b)

== system TricopterModel/3 Copter Complete/Mass Properties ==
  Arms DCMs : Inport
  CG_0 : Inport  Port=2
  m_0 : Inport  Port=3
  m : Inport  Port=4
  m_M : Inport  Port=5
  I_BAC_0 : Inport  Port=6
  Arm Inertia : MATLAB Function  TreatAsAtomicUnit=on
  Bus Selector : BusSelector  OutputSignals=T_FaFb1,T_FaFb2,T_FaFb3
  CG position : Sum
  Divide : Product  Inputs=*/
  Divide1 : Product  Inputs=**
  Divide2 : Product  Inputs=/*
  Divide3 : Product  Inputs=**
  Motors Pos sum : Sum  Inputs=+++
  Total I_BAC : Sum
  I_BAC : Outport
  CG : Outport  Port=2
  wires:
  Arms DCMs/1 -> Bus Selector/1
  Bus Selector/3 -> Arm Inertia/3(T3_FAFb)  "<T_FaFb3>"
  Bus Selector/2 -> Arm Inertia/2(T2_FAFb)  "<T_FaFb2>"
  Bus Selector/1 -> Arm Inertia/1(T1_FAFb)  "<T_FaFb1>"
  Total I_BAC/1 -> I_BAC/1
  m_0/1 -> Divide/1
  m/1 -> Divide/2, Divide2/1
  CG_0/1 -> Divide1/1
  Divide/1 -> Divide1/2
  m_M/1 -> Divide2/2
  CG position/1 -> CG/1
  Divide1/1 -> CG position/1
  Motors Pos sum/1 -> Divide3/1
  Divide2/1 -> Divide3/2
  Divide3/1 -> CG position/2
  Arm Inertia/3(r2_M) -> Motors Pos sum/2
  Arm Inertia/4(r3_M) -> Motors Pos sum/1
  Arm Inertia/1(I_M) -> Total I_BAC/2
  I_BAC_0/1 -> Total I_BAC/1
  Arm Inertia/2(r1_M) -> Motors Pos sum/3

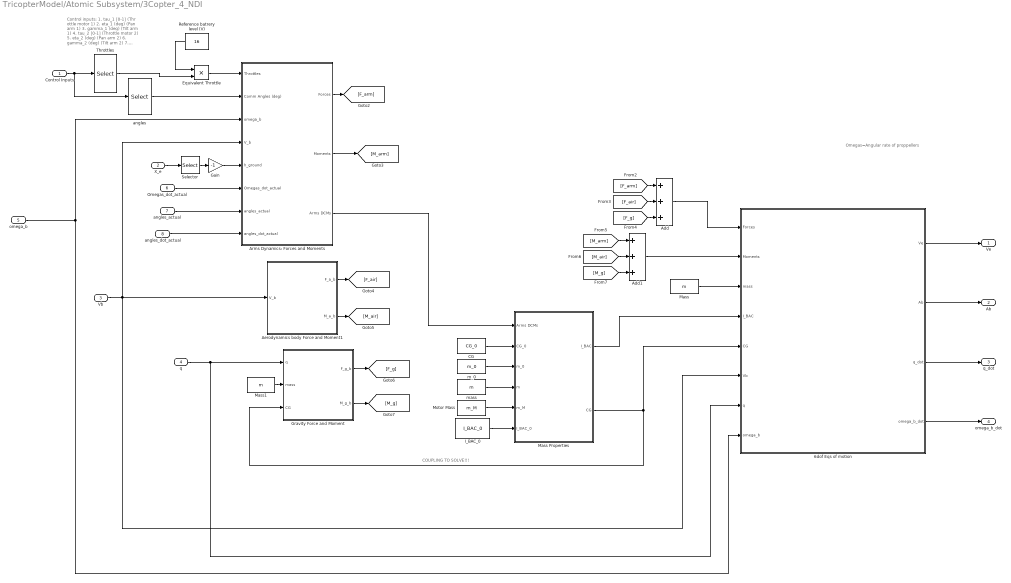
== system TricopterModel/Atomic Subsystem/3Copter_4_NDI ==
  note: COUPLING TO SOLVE!!!
  note: Omegas=Angular rate of proppellers
  note: Control inputs:
      | 1. tau_1 [0-1] (Thr ottle motor 1)
      | 2. eta_1 (deg)  (Pan arm 1)
      | 3. gamma_1 (deg)  (Tilt arm 1)
      |
      | 4. tau_2 [0-1] (Throttle motor 2)
      | 5. eta_2 (deg)  (Pan arm 2)
      | 6. gamma_2 (deg)  (Tilt arm 2)
      |
      | 7. tau_3 [0-1] (Throttle motor 3)
      | 8. eta_3 (deg)  (Pan arm  3)
      | 9. gamma_3 (deg)  (Tilt arm 3)
  Control Inputs : Inport
  X_e : Inport  Port=2
  Vb : Inport  Port=3
  q : Inport  Port=4
  omega_b : Inport  Port=5
  Omegas_dot_actual : Inport  Port=6
  angles_actual : Inport  Port=7
  angles_dot_actual : Inport  Port=8
  6dof Eqs of motion : Subsystem  TreatAsAtomicUnit=on
  Add : Sum  Inputs=+++
  Add1 : Sum  Inputs=+++
  Aerodynamics body Force and Moment1 : MATLAB Function  TreatAsAtomicUnit=on
  Arms Dynamics: Forces and Moments : Subsystem
  CG : Constant  Value=CG_0
  Equivalent Throttle : Product  Inputs=**
  Gain : Gain  Gain=-1
  Gravity Force and Moment : MATLAB Function  TreatAsAtomicUnit=on
  I_BAC_0 : Constant  Value=I_BAC_0
  Mass : Constant  Value=m
  Mass Properties : Subsystem  TreatAsAtomicUnit=on
  Mass1 : Constant  Value=m
  Motor Mass : Constant  Value=m_M
  Reference batrery level (V) : Constant  Value=16
  Selector : Selector  IndexMode=Zero-based  InputPortWidth=3  Indices=2
  Throttles : Selector  IndexMode=Zero-based  InputPortWidth=9  Indices=[0,3,6]
  "angles " : Selector  IndexMode=Zero-based  InputPortWidth=9  Indices=[1,2,4,5,7,8]
  m_0 : Constant  Value=m_0
  mass : Constant  Value=m
  Ve : Outport
  Ab : Outport  Port=2
  q_dot : Outport  Port=3
  omega_b_dot : Outport  Port=4
  wires:
  Mass/1 -> 6dof Eqs of motion/3(mass)
  Vb/1 -> Arms Dynamics: Forces and Moments/4(V_b), Aerodynamics body Force and Moment1/1(V_b), 6dof Eqs of motion/6(Vb)
  omega_b/1 -> Arms Dynamics: Forces and Moments/3(omega_b), 6dof Eqs of motion/8(omega_b)
  Mass1/1 -> Gravity Force and Moment/2(mass)
  X_e/1 -> Selector/1
  Selector/1 -> Gain/1
  Gain/1 -> Arms Dynamics: Forces and Moments/5(h_ground)
  Arms Dynamics: Forces and Moments/1(Forces) -> [F_arm]
  Arms Dynamics: Forces and Moments/2(Moments) -> [M_arm]
  Aerodynamics body Force and Moment1/1(F_a_b) -> [F_air]
  Aerodynamics body Force and Moment1/2(M_a_b) -> [M_air]
  Gravity Force and Moment/1(F_g_b) -> [F_g]
  Gravity Force and Moment/2(M_g_b) -> [M_g]
  [F_arm] -> Add/1
  [F_air] -> Add/2
  [F_g] -> Add/3
  [M_arm] -> Add1/1
  [M_g] -> Add1/3
  [M_air] -> Add1/2
  Throttles/1 -> Equivalent Throttle/2
  Control Inputs/1 -> Throttles/1, "angles "/1
  "angles "/1 -> Arms Dynamics: Forces and Moments/2(Comm Angles (deg))
  Arms Dynamics: Forces and Moments/3(Arms DCMs) -> Mass Properties/1(Arms DCMs)
  CG/1 -> Mass Properties/2(CG_0)
  Motor Mass/1 -> Mass Properties/5(m_M)
  I_BAC_0/1 -> Mass Properties/6(I_BAC_0)
  m_0/1 -> Mass Properties/3(m_0)
  mass/1 -> Mass Properties/4(m)
  Add/1 -> 6dof Eqs of motion/1(Forces)
  Mass Properties/2(CG) -> Gravity Force and Moment/3(CG), 6dof Eqs of motion/5(CG)
  Mass Properties/1(I_BAC) -> 6dof Eqs of motion/4(I_BAC)
  Equivalent Throttle/1 -> Arms Dynamics: Forces and Moments/1(Throttles)
  Reference batrery level (V)/1 -> Equivalent Throttle/1
  Add1/1 -> 6dof Eqs of motion/2(Moments)
  6dof Eqs of motion/1(Ve) -> Ve/1
  6dof Eqs of motion/2(Ab) -> Ab/1
  6dof Eqs of motion/3("q_dot ") -> q_dot/1
  6dof Eqs of motion/4(omega_b_dot) -> omega_b_dot/1
  q/1 -> 6dof Eqs of motion/7(q), Gravity Force and Moment/1(q)
  Omegas_dot_actual/1 -> Arms Dynamics: Forces and Moments/6(Omegas_dot_actual)
  angles_dot_actual/1 -> Arms Dynamics: Forces and Moments/8(angles_dot_actual)
  angles_actual/1 -> Arms Dynamics: Forces and Moments/7(angles_actual)

== system TricopterModel/Atomic Subsystem/Normalize Quaternion ==
  q : Inport
  Demux : Demux
  Math Function : Math  Operator=reciprocal  SaturateOnIntegerOverflow=on
  Mux : Mux
  Product{,1..3} (4 alike) : Product  Inputs=**
  Quaternion Modulus : aerolibutil/Quaternion Modulus
  normal(q) : Outport
  wires:
  Product3/1 -> Mux/4
  Product2/1 -> Mux/3
  Product1/1 -> Mux/2
  Product/1 -> Mux/1
  Quaternion Modulus/1 -> Math Function/1
  q/1 -> Demux/1, Quaternion Modulus/1
  Mux/1 -> normal(q)/1
  Demux/1 -> Product/1
  Demux/2 -> Product1/1
  Demux/3 -> Product2/1
  Demux/4 -> Product3/1
  Math Function/1 -> Product3/2, Product2/2, Product/2, Product1/2

== system TricopterModel/3 Copter Complete/6dof Eqs of motion/DCM1 ==
  Euler : Inport  PortDimensions=3
  Fcn11 : Fcn  Expr=u(5)*u(4)
  Fcn12 : Fcn  Expr=u(5)*u(1)
  Fcn13 : Fcn  Expr=-u(2)
  Fcn21 : Fcn  Expr=u(3)*u(2)*u(4) - u(6)*u(1)
  Fcn22 : Fcn  Expr=u(3)*u(2)*u(1) + u(6)*u(4)
  Fcn23 : Fcn  Expr=u(3)*u(5)
  Fcn31 : Fcn  Expr=u(6)*u(2)*u(4) + u(3)*u(1)
  Fcn32 : Fcn  Expr=u(6)*u(2)*u(1) - u(3)*u(4)
  Fcn33 : Fcn  Expr=u(6)*u(5)
  Mux : Mux  Inputs=2
  Mux1 : Mux  Inputs=9
  Reshape : Reshape  OutputDimensionality=Customize  OutputDimensions=[3,3]
  sincos : Trigonometry  Operator=sincos
  DCM : Outport  PortDimensions=[3,3]
  wires:
  Fcn33/1 -> Mux1/9
  Fcn32/1 -> Mux1/8
  Fcn23/1 -> Mux1/6
  Fcn22/1 -> Mux1/5
  Fcn31/1 -> Mux1/7
  Fcn21/1 -> Mux1/4
  Fcn13/1 -> Mux1/3
  Fcn12/1 -> Mux1/2
  Fcn11/1 -> Mux1/1
  Mux/1 -> Fcn22/1, Fcn23/1, Fcn31/1, Fcn33/1, Fcn32/1, Fcn21/1, Fcn13/1, Fcn12/1, Fcn11/1
  sincos/2 -> Mux/2
  sincos/1 -> Mux/1
  Reshape/1 -> DCM/1
  Euler/1 -> sincos/1
  Mux1/1 -> Reshape/1

== system TricopterModel/3 Copter Complete/6dof Eqs of motion/Normalize 4D vector ==
  v : Inport
  4D vec norm : XXCopter/4D vec norm
  Bias : Bias  Bias=eps
  Demux : Demux
  Math Function : Math  Operator=reciprocal  SaturateOnIntegerOverflow=on
  Mux : Mux
  Product{1..4} (4 alike) : Product  Inputs=**
  normal(v) : Outport
  wires:
  Bias/1 -> Math Function/1
  Product1/1 -> Mux/3
  Math Function/1 -> Product4/2, Product1/2, Product3/2, Product2/2
  Demux/3 -> Product1/1
  Product3/1 -> Mux/2
  Product2/1 -> Mux/1
  4D vec norm/1 -> Bias/1
  v/1 -> 4D vec norm/1, Demux/1
  Mux/1 -> normal(v)/1
  Demux/1 -> Product2/1
  Demux/2 -> Product3/1
  Demux/4 -> Product4/1
  Product4/1 -> Mux/4

== system TricopterModel/3 Copter Complete/6dof Eqs of motion/q_dot ==
  note: Both of these methods to compute q_dot are very similar
  omega_b : Inport
  q : Inport  Port=2
  Quaternion_dot : MATLAB Function  TreatAsAtomicUnit=on  VariantControl=Variant
  chose which method : ManualSwitch  CurrentSetting=0
  qdot : aerolib6dofsys/DCM & Euler Angles (Quaternion)/qdot  Commented=on
  q_dot : Outport
  wires:
  omega_b/1 -> Quaternion_dot/1(omega_b), qdot/1  "omega_b"
  q/1 -> Quaternion_dot/2(q), qdot/2  "q"
  chose which method/1 -> q_dot/1
  qdot/1 -> chose which method/1
  Quaternion_dot/1(q_dot) -> chose which method/2

== system TricopterModel/3 Copter Complete/Arms Dynamics: Forces and Moments/Arm Dynamics ==
  note: Motor-Propeller Coupling: Propeller Torque
  Throttle [0-1] : Inport
  Comm Angles (rad) : Inport  Port=2
  Omega_Initial : Inport  Port=3
  h_ground : Inport  Port=4
  omega_b : Inport  Port=5
  V_b : Inport  Port=6
  Aerodynamics Propeller : Subsystem  TreatAsAtomicUnit=on  mask{Rot_sign=Rot_sign}
      mask prompts: Rot_sign "Rotation Sign"
      settings: MinAlgLoopOccurrences=on
      mask TypeOptions Rot_sign: Rotation_sign/Value
  Arms Kinematics : XXCopter/Arms Kinematics  Arm_number=arm_num  Arm_hub_position=arm_hub_pos  eta_dir=eta_dir  gamma_dir=gamma_dir  h_prop=h
  Cross Product : vrlib/Utilities/Cross Product
  ESC+Motor Dynamcis : XXCopter/ESC+Motor Dynamcis  Inertia_swithc_var=Motor+Prop  J_T=J_T  tau=tau
  Ground : Ground
  Gyroscopic Moments : XXCopter/Gyroscopic Moments  Arm_axis=[l_arm;0;0]  Rot_sign=Rot_sign  eta_dir=eta_dir  gamma_dir=gamma_dir  J_T=J_T  J_FA=J_FA
  Initial_torque : Memory  X0=Torq_ini
  Servos Dynamics : XXCopter/Servos Dynamics  omega_n=omega_n  xi=xi  derv_param=c  init_eta=init_eta  init_gamma=0
  Total moments : Sum
  V^A (m/s) : Sum  Inputs=+++
  initial_omega : Memory  X0=Omega_ini
  omega_A : Sum
  omega_b1 : InportShadow  Port=5
  Forces : Outport
  Moments : Outport  Port=2
  Omega_out : Outport  Port=3
  Omega_dot_out : Outport  Port=4
  T_FaFb : Outport  Port=5
  Angles (rad) : Outport  Port=6
  r_p : Outport  Port=7
  wires:
  initial_omega/1 -> ESC+Motor Dynamcis/2
  Initial_torque/1 -> ESC+Motor Dynamcis/4
  Aerodynamics Propeller/1(Prop_Torque_out) -> Initial_torque/1
  Total moments/1 -> Moments/1
  Gyroscopic Moments/1 -> Total moments/2
  Aerodynamics Propeller/3(Moments_prop @Fb) -> Total moments/1
  Ground/1 -> Servos Dynamics/2
  Servos Dynamics/3 -> Gyroscopic Moments/5
  omega_A/1 -> Gyroscopic Moments/2
  omega_b1/1 -> omega_A/2, Gyroscopic Moments/3
  Arms Kinematics/4 -> omega_A/1
  Servos Dynamics/2 -> Arms Kinematics/2, Gyroscopic Moments/4
  Aerodynamics Propeller/2(Forces_prop @Fb) -> Forces/1
  Arms Kinematics/1 -> r_p/1, Cross Product/2, Aerodynamics Propeller/3(r_p)
  Arms Kinematics/3 -> T_FaFb/1, Aerodynamics Propeller/5(T_FaFb), Gyroscopic Moments/1
  V^A (m/s)/1 -> Aerodynamics Propeller/4(V^A)
  Arms Kinematics/2 -> V^A (m/s)/3
  V_b/1 -> V^A (m/s)/1
  Cross Product/1 -> V^A (m/s)/2
  omega_b/1 -> Cross Product/1
  Servos Dynamics/1 -> Angles (rad)/1, Arms Kinematics/1
  Comm Angles (rad)/1 -> Servos Dynamics/1
  h_ground/1 -> Aerodynamics Propeller/2(h_ground)
  ESC+Motor Dynamcis/1 -> Aerodynamics Propeller/1(Omega), Omega_out/1, Gyroscopic Moments/6, initial_omega/1  "Omega"
  ESC+Motor Dynamcis/2 -> Omega_dot_out/1, Gyroscopic Moments/7  "Omega_dot"
  Omega_Initial/1 -> ESC+Motor Dynamcis/3
  Throttle [0-1]/1 -> ESC+Motor Dynamcis/1

== system TricopterModel/3 Copter Complete/Arms Dynamics: Forces and Moments/Arm Dynamics1 ==
  note: Motor-Propeller Coupling: Propeller Torque
  Throttle [0-1] : Inport
  Comm Angles (rad) : Inport  Port=2
  Omega_Initial : Inport  Port=3
  h_ground : Inport  Port=4
  omega_b : Inport  Port=5
  V_b : Inport  Port=6
  Aerodynamics Propeller : Subsystem  TreatAsAtomicUnit=on  mask{Rot_sign=Rot_sign}
      mask prompts: Rot_sign "Rotation Sign"
      settings: MinAlgLoopOccurrences=on
      mask TypeOptions Rot_sign: Rotation_sign/Value
  Arms Kinematics : XXCopter/Arms Kinematics  Arm_number=arm_num  Arm_hub_position=arm_hub_pos  eta_dir=eta_dir  gamma_dir=gamma_dir  h_prop=h
  Cross Product : vrlib/Utilities/Cross Product
  ESC+Motor Dynamcis : XXCopter/ESC+Motor Dynamcis  Inertia_swithc_var=Motor+Prop  J_T=J_T  tau=tau
  Ground : Ground
  Gyroscopic Moments : XXCopter/Gyroscopic Moments  Arm_axis=[0;l_arm;0]  Rot_sign=Rot_sign  eta_dir=eta_dir  gamma_dir=gamma_dir  J_T=J_T  J_FA=J_FA
  Initial_torque : Memory  X0=Torq_ini
  Servos Dynamics : XXCopter/Servos Dynamics  omega_n=omega_n  xi=xi  derv_param=c  init_eta=init_eta  init_gamma=0
  Total moments : Sum
  V^A (m/s) : Sum  Inputs=+++
  initial_omega : Memory  X0=Omega_ini
  omega_A : Sum
  omega_b1 : InportShadow  Port=5
  Forces : Outport
  Moments : Outport  Port=2
  Omega_out : Outport  Port=3
  Omega_dot_out : Outport  Port=4
  T_FaFb : Outport  Port=5
  Angles (rad) : Outport  Port=6
  r_p : Outport  Port=7
  wires:
  initial_omega/1 -> ESC+Motor Dynamcis/2
  Initial_torque/1 -> ESC+Motor Dynamcis/4
  Aerodynamics Propeller/1(Prop_Torque_out) -> Initial_torque/1
  Total moments/1 -> Moments/1
  Gyroscopic Moments/1 -> Total moments/2
  Aerodynamics Propeller/3(Moments_prop @Fb) -> Total moments/1
  Ground/1 -> Servos Dynamics/2
  Servos Dynamics/3 -> Gyroscopic Moments/5
  omega_A/1 -> Gyroscopic Moments/2
  omega_b1/1 -> omega_A/2, Gyroscopic Moments/3
  Arms Kinematics/4 -> omega_A/1
  Servos Dynamics/2 -> Arms Kinematics/2, Gyroscopic Moments/4
  Aerodynamics Propeller/2(Forces_prop @Fb) -> Forces/1
  Arms Kinematics/1 -> r_p/1, Cross Product/2, Aerodynamics Propeller/3(r_p)
  Arms Kinematics/3 -> T_FaFb/1, Aerodynamics Propeller/5(T_FaFb), Gyroscopic Moments/1
  V^A (m/s)/1 -> Aerodynamics Propeller/4(V^A)
  Arms Kinematics/2 -> V^A (m/s)/3
  V_b/1 -> V^A (m/s)/1
  Cross Product/1 -> V^A (m/s)/2
  omega_b/1 -> Cross Product/1
  Servos Dynamics/1 -> Angles (rad)/1, Arms Kinematics/1
  Comm Angles (rad)/1 -> Servos Dynamics/1
  h_ground/1 -> Aerodynamics Propeller/2(h_ground)
  ESC+Motor Dynamcis/1 -> Aerodynamics Propeller/1(Omega), Omega_out/1, Gyroscopic Moments/6, initial_omega/1  "Omega"
  ESC+Motor Dynamcis/2 -> Omega_dot_out/1, Gyroscopic Moments/7  "Omega_dot"
  Omega_Initial/1 -> ESC+Motor Dynamcis/3
  Throttle [0-1]/1 -> ESC+Motor Dynamcis/1

== system TricopterModel/3 Copter Complete/Arms Dynamics: Forces and Moments/Arm Dynamics2 ==
  note: Motor-Propeller Coupling: Propeller Torque
  Throttle [0-1] : Inport
  Comm Angles (rad) : Inport  Port=2
  Omega_Initial : Inport  Port=3
  h_ground : Inport  Port=4
  omega_b : Inport  Port=5
  V_b : Inport  Port=6
  Aerodynamics Propeller : Subsystem  TreatAsAtomicUnit=on  mask{Rot_sign=Rot_sign}
      mask prompts: Rot_sign "Rotation Sign"
      settings: MinAlgLoopOccurrences=on
      mask TypeOptions Rot_sign: Rotation_sign/Value
  Arms Kinematics : XXCopter/Arms Kinematics  Arm_number=arm_num  Arm_hub_position=arm_hub_pos  eta_dir=eta_dir  gamma_dir=gamma_dir  h_prop=h
  Cross Product : vrlib/Utilities/Cross Product
  ESC+Motor Dynamcis : XXCopter/ESC+Motor Dynamcis  Inertia_swithc_var=Motor+Prop  J_T=J_T  tau=tau
  Ground : Ground
  Gyroscopic Moments : XXCopter/Gyroscopic Moments  Arm_axis=[0;-l_arm;0]  Rot_sign=Rot_sign  eta_dir=eta_dir  gamma_dir=gamma_dir  J_T=J_T  J_FA=J_FA
  Initial_torque : Memory  X0=Torq_ini
  Servos Dynamics : XXCopter/Servos Dynamics  omega_n=omega_n  xi=xi  derv_param=c  init_eta=init_eta  init_gamma=0
  Total moments : Sum
  V^A (m/s) : Sum  Inputs=+++
  initial_omega : Memory  X0=Omega_ini
  omega_A : Sum
  omega_b1 : InportShadow  Port=5
  Forces : Outport
  Moments : Outport  Port=2
  Omega_out : Outport  Port=3
  Omega_dot_out : Outport  Port=4
  T_FaFb : Outport  Port=5
  Angles (rad) : Outport  Port=6
  r_p : Outport  Port=7
  wires:
  initial_omega/1 -> ESC+Motor Dynamcis/2
  Initial_torque/1 -> ESC+Motor Dynamcis/4
  Aerodynamics Propeller/1(Prop_Torque_out) -> Initial_torque/1
  Total moments/1 -> Moments/1
  Gyroscopic Moments/1 -> Total moments/2
  Aerodynamics Propeller/3(Moments_prop @Fb) -> Total moments/1
  Ground/1 -> Servos Dynamics/2
  Servos Dynamics/3 -> Gyroscopic Moments/5
  omega_A/1 -> Gyroscopic Moments/2
  omega_b1/1 -> omega_A/2, Gyroscopic Moments/3
  Arms Kinematics/4 -> omega_A/1
  Servos Dynamics/2 -> Arms Kinematics/2, Gyroscopic Moments/4
  Aerodynamics Propeller/2(Forces_prop @Fb) -> Forces/1
  Arms Kinematics/1 -> r_p/1, Cross Product/2, Aerodynamics Propeller/3(r_p)
  Arms Kinematics/3 -> T_FaFb/1, Aerodynamics Propeller/5(T_FaFb), Gyroscopic Moments/1
  V^A (m/s)/1 -> Aerodynamics Propeller/4(V^A)
  Arms Kinematics/2 -> V^A (m/s)/3
  V_b/1 -> V^A (m/s)/1
  Cross Product/1 -> V^A (m/s)/2
  omega_b/1 -> Cross Product/1
  Servos Dynamics/1 -> Angles (rad)/1, Arms Kinematics/1
  Comm Angles (rad)/1 -> Servos Dynamics/1
  h_ground/1 -> Aerodynamics Propeller/2(h_ground)
  ESC+Motor Dynamcis/1 -> Aerodynamics Propeller/1(Omega), Omega_out/1, Gyroscopic Moments/6, initial_omega/1  "Omega"
  ESC+Motor Dynamcis/2 -> Omega_dot_out/1, Gyroscopic Moments/7  "Omega_dot"
  Omega_Initial/1 -> ESC+Motor Dynamcis/3
  Throttle [0-1]/1 -> ESC+Motor Dynamcis/1

== system TricopterModel/Atomic Subsystem/3Copter_4_NDI/6dof Eqs of motion ==
  Forces : Inport
  Moments : Inport  Port=2
  mass : Inport  Port=3
  I_BAC : Inport  Port=4
  CG : Inport  Port=5
  Vb : Inport  Port=6
  q : Inport  Port=7
  omega_b : Inport  Port=8
  Normalize Quaternion : Subsystem  TreatAsAtomicUnit=on
  Position Eqs : MATLAB Function  TreatAsAtomicUnit=on
  Rotational eqs : MATLAB Function  TreatAsAtomicUnit=on
  SV_F_b_to_SV_FI : MATLAB Function  TreatAsAtomicUnit=on
  q_dot : Subsystem  TreatAsAtomicUnit=on
  Ve : Outport
  Ab : Outport  Port=2
  "q_dot " : Outport  Port=3
  omega_b_dot : Outport  Port=4
  wires:
  I_BAC/1 -> Rotational eqs/3(I_BAC)
  mass/1 -> Position Eqs/5(m)
  Forces/1 -> Position Eqs/4(Forces)
  omega_b/1 -> Position Eqs/2(omega_b), q_dot/1(omega_b), Rotational eqs/1(omega_b)
  Rotational eqs/1(omega_dot) -> omega_b_dot/1, Position Eqs/3(omega_b_dot)
  Position Eqs/1(A_b) -> Ab/1  "A_b"
  CG/1 -> Position Eqs/6(CG)
  q_dot/1(q_dot) -> "q_dot "/1
  SV_F_b_to_SV_FI/1(V_e) -> Ve/1
  Moments/1 -> Rotational eqs/2(Moments)
  Vb/1 -> SV_F_b_to_SV_FI/2(V_b), Position Eqs/1(Vb)
  q/1 -> Normalize Quaternion/1(q)
  Normalize Quaternion/1(normal(q)) -> SV_F_b_to_SV_FI/1(q), q_dot/2(q)
